simulink model "inverted_pendulum"  (R2021a)
settings: Solver=VariableStepAuto  StartTime=0.0  StopTime=20  MaxStep=0.01  RelTol=1e-3
undefined symbols (not defined in the file): A, alpha, B, beta, bm, bp, C_acc, C_acc_double_enc, C_acc_enc, dt, g, ideal_acc_height, J1, Jw, K, Ke, Kt, L1, L_acc, L_acc_double_enc, L_acc_enc, La, Ra, real_acc_height, V_nom, wn, x0
(part 1 of 2)
settings Model: Creator=jpss8  LastModifiedBy=jpss8

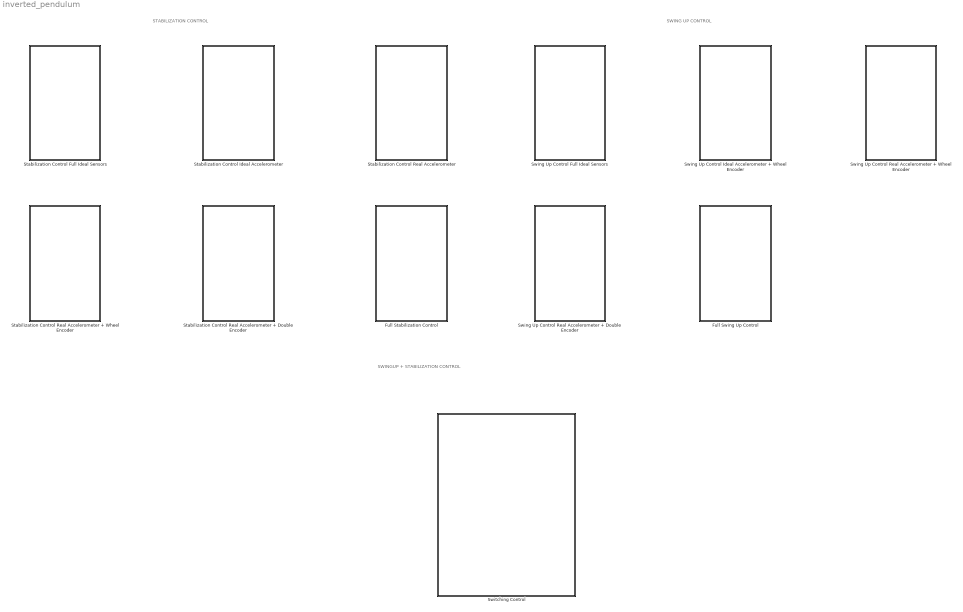
== system inverted_pendulum ==
  note: STABILIZATION CONTROL
  note: SWING UP CONTROL
  note: SWINGUP + STABILIZATION CONTROL
  Full Stabilization Control : Subsystem
  Full Swing Up Control : Subsystem
  Stabilization Control Full Ideal Sensors : Subsystem
  "Stabilization Control Ideal Accelerometer " : Subsystem
  Stabilization Control Real Accelerometer : Subsystem
  Stabilization Control Real Accelerometer + Double Encoder : Subsystem
  Stabilization Control Real Accelerometer + Wheel Encoder : Subsystem
  Swing Up Control Full Ideal Sensors : Subsystem
  Swing Up Control Ideal Accelerometer + Wheel Encoder : Subsystem
  Swing Up Control Real Accelerometer + Double Encoder : Subsystem
  Swing Up Control Real Accelerometer + Wheel Encoder : Subsystem
  Switching Control : Subsystem

== system inverted_pendulum/Full Stabilization Control ==
  note: DC Motor Saturation
  LQR Controller : Subsystem
  Nonlinear Inverted Pendulum : Subsystem
  Real Sensors : Subsystem
  Signal Processing : Subsystem
  State Estimation : Subsystem
  Vmax = 24V : Saturate  UpperLimit=V_nom  LowerLimit=-V_nom
  wires:
  Vmax = 24V/1 -> Nonlinear Inverted Pendulum/1(V), State Estimation/1(V)
  LQR Controller/1(V) -> Vmax = 24V/1
  Real Sensors/1(Acc) -> Signal Processing/4(Acc)
  Real Sensors/2(Gyro) -> Signal Processing/3(Gyro)
  Signal Processing/1(Measured States) -> State Estimation/2(Measured States)
  Nonlinear Inverted Pendulum/1(NL Full State + d2theta) -> Real Sensors/1(NL Full State + d2theta)
  Real Sensors/3(wm) -> Signal Processing/2(wm)
  Real Sensors/4(wp) -> Signal Processing/1(wp)

== system inverted_pendulum/Full Swing Up Control ==
  note: DC Motor Saturation
  Bang Bang Energy Controller : Subsystem
  Ideal Sensors : Subsystem
  Nonlinear Inverted Pendulum : Subsystem
  Vmax = 24V : Saturate  UpperLimit=V_nom  LowerLimit=-V_nom
  wires:
  Vmax = 24V/1 -> Nonlinear Inverted Pendulum/1(V)
  Bang Bang Energy Controller/1(V) -> Vmax = 24V/1
  Nonlinear Inverted Pendulum/1(NL Full State) -> Ideal Sensors/1(Full State)

== system inverted_pendulum/Stabilization Control Full Ideal Sensors ==
  note: DC Motor Saturation
  Ideal Sensors : Subsystem
  LQR Controller : Subsystem
  Nonlinear Inverted Pendulum : Subsystem
  Scope : Scope
  Vmax = 24V : Saturate  UpperLimit=V_nom  LowerLimit=-V_nom
  wires:
  Vmax = 24V/1 -> Nonlinear Inverted Pendulum/1(V)
  LQR Controller/1(V) -> Vmax = 24V/1
  Nonlinear Inverted Pendulum/1(NL Full State) -> Scope/1, Ideal Sensors/1(Full State)
  Ideal Sensors/1(Measured States) -> LQR Controller/1(Measured Full State)

== system inverted_pendulum/Stabilization Control Ideal Accelerometer  ==
  note: DC Motor Saturation
  LQR Controller : Subsystem
  Nonlinear Inverted Pendulum : Subsystem
  Sensors : Subsystem
  Signal Processing : Subsystem
  State Estimation : Subsystem
  Vmax = 24V : Saturate  UpperLimit=V_nom  LowerLimit=-V_nom
  wires:
  Vmax = 24V/1 -> Nonlinear Inverted Pendulum/1(V), State Estimation/1(V)
  LQR Controller/1(V) -> Vmax = 24V/1
  Sensors/1(Acc) -> Signal Processing/1(Acc)
  Signal Processing/1(Measured States) -> State Estimation/2(Measured States)
  Nonlinear Inverted Pendulum/1(NL Full State + d2theta) -> Sensors/1(NL Full State)

== system inverted_pendulum/Stabilization Control Real Accelerometer ==
  note: DC Motor Saturation
  LQR Controller : Subsystem
  Nonlinear Inverted Pendulum : Subsystem
  Sensors : Subsystem
  Signal Processing1 : Subsystem
  State Estimation : Subsystem
  Vmax = 24V : Saturate  UpperLimit=V_nom  LowerLimit=-V_nom
  wires:
  Vmax = 24V/1 -> Nonlinear Inverted Pendulum/1(V), State Estimation/1(V)
  LQR Controller/1(V) -> Vmax = 24V/1
  Sensors/1(Acc) -> Signal Processing1/2(Acc)
  Signal Processing1/1(Measured States) -> State Estimation/2(Measured States)
  Nonlinear Inverted Pendulum/1(NL Full State + d2theta) -> Sensors/1(NL Full State)
  Sensors/2(Gyro) -> Signal Processing1/1(Gyro)

== system inverted_pendulum/Stabilization Control Real Accelerometer + Double Encoder ==
  note: DC Motor Saturation
  LQR Controller : Subsystem
  Nonlinear Inverted Pendulum : Subsystem
  Real Sensors : Subsystem
  Signal Processing : Subsystem
  State Estimation : Subsystem
  Vmax = 24V : Saturate  UpperLimit=V_nom  LowerLimit=-V_nom
  wires:
  Vmax = 24V/1 -> Nonlinear Inverted Pendulum/1(V), State Estimation/1(V)
  LQR Controller/1(V) -> Vmax = 24V/1
  Real Sensors/1(Acc) -> Signal Processing/4(Acc)
  Real Sensors/2(Gyro) -> Signal Processing/3(Gyro)
  Signal Processing/1(Measured States) -> State Estimation/2(Measured States)
  Nonlinear Inverted Pendulum/1(NL Full State + d2theta) -> Real Sensors/1(NL Full State + d2theta)
  Real Sensors/3(wm) -> Signal Processing/2(wm)
  Real Sensors/4(wp) -> Signal Processing/1(wp)

== system inverted_pendulum/Stabilization Control Real Accelerometer + Wheel Encoder ==
  note: DC Motor Saturation
  LQR Controller : Subsystem
  Nonlinear Inverted Pendulum : Subsystem
  Real Sensors : Subsystem
  Signal Processing : Subsystem
  State Estimation : Subsystem
  Vmax = 24V : Saturate  UpperLimit=V_nom  LowerLimit=-V_nom
  wires:
  Vmax = 24V/1 -> Nonlinear Inverted Pendulum/1(V), State Estimation/1(V)
  LQR Controller/1(V) -> Vmax = 24V/1
  Real Sensors/1(Acc) -> Signal Processing/3(Acc)
  Real Sensors/2(Gyro) -> Signal Processing/2(Gyro)
  Signal Processing/1(Measured States) -> State Estimation/2(Measured States)
  Nonlinear Inverted Pendulum/1(NL Full State + d2theta) -> Real Sensors/1(NL Full State)
  Real Sensors/3(wm) -> Signal Processing/1(wm)

== system inverted_pendulum/Swing Up Control Full Ideal Sensors ==
  note: DC Motor Saturation
  Bang Bang Energy Controller : Subsystem
  Demux : Demux
  Ideal Sensors : Subsystem
  Nonlinear Inverted Pendulum : Subsystem
  Scope : Scope
  Scope1 : Scope
  Scope2 : Scope
  Vmax = 24V : Saturate  UpperLimit=V_nom  LowerLimit=-V_nom
  wires:
  Vmax = 24V/1 -> Scope2/1, Nonlinear Inverted Pendulum/1(V)
  Bang Bang Energy Controller/1(V) -> Vmax = 24V/1
  Nonlinear Inverted Pendulum/1(NL Full State) -> Demux/1, Ideal Sensors/1(Full State)
  Demux/1 -> Scope/1
  Demux/3 -> Scope1/1

== system inverted_pendulum/Swing Up Control Ideal Accelerometer + Wheel Encoder ==
  note: DC Motor Saturation
  Bang Bang Energy Controller : Subsystem
  Ideal Sensors : Subsystem
  Nonlinear Inverted Pendulum : Subsystem
  Vmax = 24V : Saturate  UpperLimit=V_nom  LowerLimit=-V_nom
  wires:
  Vmax = 24V/1 -> Nonlinear Inverted Pendulum/1(V)
  Bang Bang Energy Controller/1(V) -> Vmax = 24V/1
  Nonlinear Inverted Pendulum/1(NL Full State) -> Ideal Sensors/1(Full State)

== system inverted_pendulum/Swing Up Control Real Accelerometer + Double Encoder ==
  note: DC Motor Saturation
  Bang Bang Energy Controller : Subsystem
  Ideal Sensors : Subsystem
  Nonlinear Inverted Pendulum : Subsystem
  Vmax = 24V : Saturate  UpperLimit=V_nom  LowerLimit=-V_nom
  wires:
  Vmax = 24V/1 -> Nonlinear Inverted Pendulum/1(V)
  Bang Bang Energy Controller/1(V) -> Vmax = 24V/1
  Nonlinear Inverted Pendulum/1(NL Full State) -> Ideal Sensors/1(Full State)

== system inverted_pendulum/Swing Up Control Real Accelerometer + Wheel Encoder ==
  note: DC Motor Saturation
  Bang Bang Energy Controller : Subsystem
  Ideal Sensors : Subsystem
  Nonlinear Inverted Pendulum : Subsystem
  Vmax = 24V : Saturate  UpperLimit=V_nom  LowerLimit=-V_nom
  wires:
  Vmax = 24V/1 -> Nonlinear Inverted Pendulum/1(V)
  Bang Bang Energy Controller/1(V) -> Vmax = 24V/1
  Nonlinear Inverted Pendulum/1(NL Full State) -> Ideal Sensors/1(Full State)

== system inverted_pendulum/Switching Control ==
  note: DC Motor Saturation
  Constant : Constant  Value=0.25
  Demux : Demux
  Demux1 : Demux
  Ideal Sensors : Subsystem
  Nonlinear Inverted Pendulum : Subsystem
  Scope : Scope  NumInputPorts=2
  Scope1 : Scope
  Switching Controller : Stateflow chart  TreatAsAtomicUnit=on
  Vmax = 24V : Saturate  UpperLimit=V_nom  LowerLimit=-V_nom
  wires:
  Vmax = 24V/1 -> Nonlinear Inverted Pendulum/1(V)
  Nonlinear Inverted Pendulum/1(NL Full State) -> Demux1/1, Ideal Sensors/1(Full State)
  Switching Controller/1(V) -> Vmax = 24V/1
  Demux/1 -> Switching Controller/1(theta)
  Demux/2 -> Switching Controller/2(wp)
  Demux/3 -> Switching Controller/3(wm)
  Demux/4 -> Switching Controller/4(ia)
  Demux1/1 -> Scope/1
  Constant/1 -> Scope/2
  Demux1/3 -> Scope1/1
  Ideal Sensors/1(Measured States) -> Demux/1

== system inverted_pendulum/Full Stabilization Control/LQR Controller ==
  Estimated Full State : Inport
  Gain : Gain  Gain=-K  Multiplication=Matrix(K*u)
  V : Outport
  wires:
  Estimated Full State/1 -> Gain/1
  Gain/1 -> V/1

== system inverted_pendulum/Full Stabilization Control/Nonlinear Inverted Pendulum ==
  V : Inport
  DC Motor + Wheel : Subsystem
  Inverted Pendulum : Subsystem
  Mux : Mux  Inputs=5
  NL Full State + d2theta : Outport
  wires:
  Mux/1 -> NL Full State + d2theta/1
  Inverted Pendulum/3(d2theta) -> Mux/5  "d2theta"
  Inverted Pendulum/2(wp) -> Mux/2  "wp"
  Inverted Pendulum/1(theta) -> Mux/1  "theta"
  DC Motor + Wheel/1(wm) -> Mux/3, Inverted Pendulum/1(wm)  "wm"
  DC Motor + Wheel/2(ia) -> Inverted Pendulum/2(ia), Mux/4  "ia"
  V/1 -> DC Motor + Wheel/1(V)

== system inverted_pendulum/Full Stabilization Control/Real Sensors ==
  NL Full State + d2theta : Inport
  Demux : Demux  Outputs=5
  IMU : Subsystem
  Pendulum Encoder : Subsystem
  Terminator : Terminator
  Wheel Encoder : Subsystem
  Acc : Outport
  Gyro : Outport  Port=2
  wm : Outport  Port=3
  wp : Outport  Port=4
  wires:
  NL Full State + d2theta/1 -> Demux/1
  Demux/1 -> IMU/1(theta)
  Demux/3 -> Wheel Encoder/1(In1)
  Demux/4 -> Terminator/1
  IMU/2(G) -> Gyro/1
  IMU/1(A) -> Acc/1
  Demux/5 -> IMU/3(d2theta)
  Wheel Encoder/1(wm) -> wm/1
  Pendulum Encoder/1(wp) -> wp/1
  Demux/2 -> IMU/2(wp), Pendulum Encoder/1(In1)

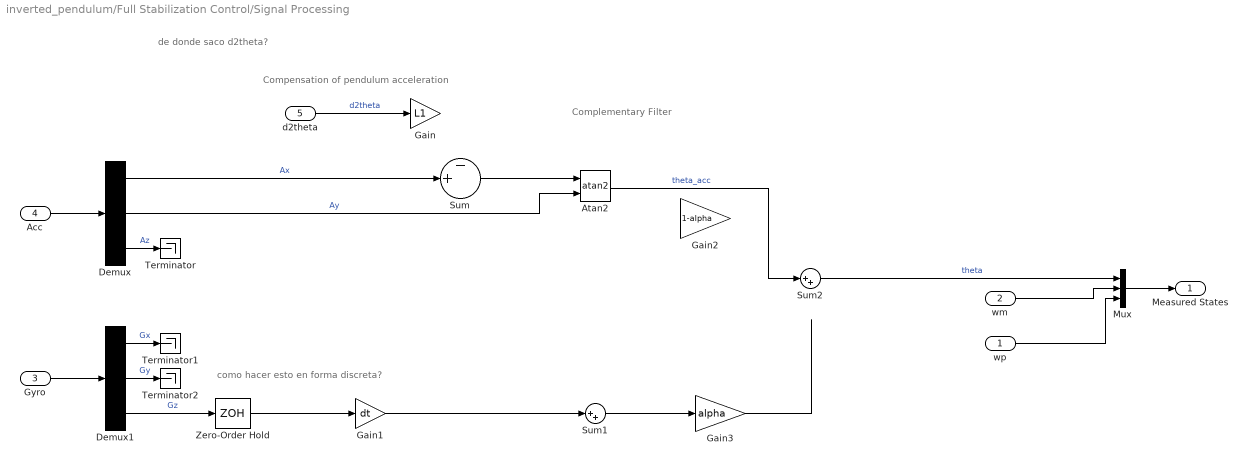
== system inverted_pendulum/Full Stabilization Control/Signal Processing ==
  note: como hacer esto en forma discreta?
  note: Complementary Filter
  note: de donde saco d2theta?
  note: Compensation of pendulum acceleration
  wp : Inport
  wm : Inport  Port=2
  Gyro : Inport  Port=3
  Acc : Inport  Port=4
  d2theta : Inport  Port=5
  Atan2 : Trigonometry  Operator=atan2
  Demux : Demux  Outputs=3
  Demux1 : Demux  Outputs=3
  Gain : Gain  Gain=L1
  Gain1 : Gain  Gain=dt
  Gain2 : Gain  Gain=1-alpha
  Gain3 : Gain  Gain=alpha
  Mux : Mux  Inputs=3
  Sum : Sum  Inputs=-+|
  Sum1 : Sum  Inputs=|++
  Sum2 : Sum  Inputs=|++
  Terminator : Terminator
  Terminator1 : Terminator
  Terminator2 : Terminator
  Zero-Order Hold : ZeroOrderHold  SampleTime=-1
  Measured States : Outport
  wires:
  Gyro/1 -> Demux1/1
  Acc/1 -> Demux/1
  Demux/1 -> Sum/2  "Ax"
  Demux/2 -> Atan2/2  "Ay"
  Demux/3 -> Terminator/1  "Az"
  Sum/1 -> Atan2/1
  d2theta/1 -> Gain/1  "d2theta"
  Atan2/1 -> Sum2/1  "theta_acc"
  Demux1/1 -> Terminator1/1  "Gx"
  Demux1/2 -> Terminator2/1  "Gy"
  Demux1/3 -> Zero-Order Hold/1  "Gz"
  Sum2/1 -> Mux/1  "theta"
  Sum1/1 -> Gain3/1
  Gain1/1 -> Sum1/1
  Zero-Order Hold/1 -> Gain1/1
  Gain3/1 -> ?
  ? -> Sum1/2
  wm/1 -> Mux/2
  Mux/1 -> Measured States/1
  wp/1 -> Mux/3

== system inverted_pendulum/Full Stabilization Control/State Estimation ==
  V : Inport
  Measured States : Inport  Port=2
  Gain : Gain  Gain=L_acc_double_enc  Multiplication=Matrix(K*u)
  Gain1 : Gain  Gain=C_acc_double_enc  Multiplication=Matrix(K*u)
  Gain2 : Gain  Gain=A  Multiplication=Matrix(K*u)
  Gain3 : Gain  Gain=B  Multiplication=Matrix(K*u)
  Integrator : Integrator
  Sum : Sum  Inputs=|+-
  Sum1 : Sum  Inputs=+++
  Estimated Full State : Outport
  wires:
  Measured States/1 -> Sum/1
  V/1 -> Gain3/1
  Integrator/1 -> Gain1/1, Gain2/1, Estimated Full State/1
  Gain3/1 -> Sum1/2
  Sum1/1 -> Integrator/1
  Gain2/1 -> Sum1/3
  Sum/1 -> Gain/1
  Gain1/1 -> Sum/2
  Gain/1 -> Sum1/1

== system inverted_pendulum/Full Swing Up Control/Bang Bang Energy Controller ==
  Measured Full State : Inport
  Demux : Demux
  Energy Calculation : Subsystem
  Gain : Gain  Gain=3.5
  Gain1 : Gain  Gain=0.5
  Gain2 : Gain  Gain=-V_nom
  Product : Product
  Scope : Scope
  Scope1 : Scope
  Sum : Sum  Inputs=|+-
  V : Outport
  wires:
  Energy Calculation/1(Eref-E) -> Scope/1, Product/1
  Measured Full State/1 -> Demux/1
  Demux/2 -> Energy Calculation/2(wp), Product/2  "wp"
  Product/1 -> Gain/1
  Gain/1 -> Sum/1
  Demux/3 -> Gain1/1  "wm"
  Gain1/1 -> Sum/2
  Sum/1 -> Gain2/1
  Demux/1 -> Energy Calculation/1(theta)
  Gain2/1 -> Scope1/1, V/1

== system inverted_pendulum/Full Swing Up Control/Ideal Sensors ==
  note: Ideal Sensors
  Full State : Inport
  Gain : Gain
  Measured States : Outport
  wires:
  Full State/1 -> Gain/1
  Gain/1 -> Measured States/1

== system inverted_pendulum/Full Swing Up Control/Nonlinear Inverted Pendulum ==
  V : Inport
  DC Motor + Wheel : Subsystem
  Inverted Pendulum : Subsystem
  Mux : Mux
  NL Full State : Outport
  wires:
  Mux/1 -> NL Full State/1
  Inverted Pendulum/2(wp) -> Mux/2  "wp"
  Inverted Pendulum/1(theta) -> Mux/1  "theta"
  DC Motor + Wheel/1(wm) -> Mux/3, Inverted Pendulum/1(wm)  "wm"
  DC Motor + Wheel/2(ia) -> Inverted Pendulum/2(ia), Mux/4  "ia"
  V/1 -> DC Motor + Wheel/1(V)

== system inverted_pendulum/Stabilization Control Full Ideal Sensors/Ideal Sensors ==
  note: Ideal Sensors
  Full State : Inport
  Gain : Gain
  Measured States : Outport
  wires:
  Full State/1 -> Gain/1
  Gain/1 -> Measured States/1

== system inverted_pendulum/Stabilization Control Full Ideal Sensors/LQR Controller ==
  Measured Full State : Inport
  Gain : Gain  Gain=-K  Multiplication=Matrix(K*u)
  V : Outport
  wires:
  Measured Full State/1 -> Gain/1
  Gain/1 -> V/1

== system inverted_pendulum/Stabilization Control Full Ideal Sensors/Nonlinear Inverted Pendulum ==
  V : Inport
  DC Motor + Wheel : Subsystem
  Inverted Pendulum : Subsystem
  Mux : Mux
  NL Full State : Outport
  wires:
  Mux/1 -> NL Full State/1
  Inverted Pendulum/2(wp) -> Mux/2  "wp"
  Inverted Pendulum/1(theta) -> Mux/1  "theta"
  DC Motor + Wheel/1(wm) -> Mux/3, Inverted Pendulum/1(wm)  "wm"
  DC Motor + Wheel/2(ia) -> Inverted Pendulum/2(ia), Mux/4  "ia"
  V/1 -> DC Motor + Wheel/1(V)

== system inverted_pendulum/Stabilization Control Ideal Accelerometer /LQR Controller ==
  Estimated Full State : Inport
  Gain : Gain  Gain=-K  Multiplication=Matrix(K*u)
  V : Outport
  wires:
  Estimated Full State/1 -> Gain/1
  Gain/1 -> V/1

== system inverted_pendulum/Stabilization Control Ideal Accelerometer /Nonlinear Inverted Pendulum ==
  V : Inport
  DC Motor + Wheel : Subsystem
  Inverted Pendulum : Subsystem
  Mux : Mux  Inputs=5
  NL Full State + d2theta : Outport
  wires:
  Mux/1 -> NL Full State + d2theta/1
  Inverted Pendulum/3(d2theta) -> Mux/5  "d2theta"
  Inverted Pendulum/2(wp) -> Mux/2  "wp"
  Inverted Pendulum/1(theta) -> Mux/1  "theta"
  DC Motor + Wheel/1(wm) -> Mux/3, Inverted Pendulum/1(wm)  "wm"
  DC Motor + Wheel/2(ia) -> Inverted Pendulum/2(ia), Mux/4  "ia"
  V/1 -> DC Motor + Wheel/1(V)

== system inverted_pendulum/Stabilization Control Ideal Accelerometer /Sensors ==
  NL Full State : Inport
  Demux : Demux  Outputs=5
  IMU : Subsystem
  Terminator : Terminator
  Terminator1 : Terminator
  Acc : Outport
  Gyro : Outport  Port=2
  wires:
  NL Full State/1 -> Demux/1
  Demux/2 -> IMU/2(wp)
  Demux/1 -> IMU/1(theta)
  Demux/4 -> Terminator/1
  IMU/2(G) -> Gyro/1
  IMU/1(A) -> Acc/1
  Demux/5 -> IMU/3(d2theta)
  Demux/3 -> Terminator1/1

== system inverted_pendulum/Stabilization Control Ideal Accelerometer /Signal Processing ==
  Acc : Inport
  Atan2 : Trigonometry  Operator=atan2
  Demux : Demux  Outputs=3
  Terminator : Terminator
  Measured States : Outport
  wires:
  Acc/1 -> Demux/1
  Demux/1 -> Atan2/1  "Ax"
  Demux/2 -> Atan2/2  "Ay"
  Demux/3 -> Terminator/1  "Az"
  Atan2/1 -> Measured States/1  "theta_acc"

== system inverted_pendulum/Stabilization Control Ideal Accelerometer /State Estimation ==
  V : Inport
  Measured States : Inport  Port=2
  Gain : Gain  Gain=L_acc  Multiplication=Matrix(K*u)
  Gain1 : Gain  Gain=C_acc  Multiplication=Matrix(K*u)
  Gain2 : Gain  Gain=A  Multiplication=Matrix(K*u)
  Gain3 : Gain  Gain=B  Multiplication=Matrix(K*u)
  Integrator : Integrator
  Sum : Sum  Inputs=|+-
  Sum1 : Sum  Inputs=+++
  Estimated Full State : Outport
  wires:
  Measured States/1 -> Sum/1
  V/1 -> Gain3/1
  Integrator/1 -> Gain1/1, Gain2/1, Estimated Full State/1
  Gain3/1 -> Sum1/2
  Sum1/1 -> Integrator/1
  Gain2/1 -> Sum1/3
  Sum/1 -> Gain/1
  Gain1/1 -> Sum/2
  Gain/1 -> Sum1/1

== system inverted_pendulum/Stabilization Control Real Accelerometer/LQR Controller ==
  Estimated Full State : Inport
  Gain : Gain  Gain=-K  Multiplication=Matrix(K*u)
  V : Outport
  wires:
  Estimated Full State/1 -> Gain/1
  Gain/1 -> V/1

== system inverted_pendulum/Stabilization Control Real Accelerometer/Nonlinear Inverted Pendulum ==
  V : Inport
  DC Motor + Wheel : Subsystem
  Inverted Pendulum : Subsystem
  Mux : Mux  Inputs=5
  NL Full State + d2theta : Outport
  wires:
  Mux/1 -> NL Full State + d2theta/1
  Inverted Pendulum/3(d2theta) -> Mux/5  "d2theta"
  Inverted Pendulum/2(wp) -> Mux/2  "wp"
  Inverted Pendulum/1(theta) -> Mux/1  "theta"
  DC Motor + Wheel/1(wm) -> Mux/3, Inverted Pendulum/1(wm)  "wm"
  DC Motor + Wheel/2(ia) -> Inverted Pendulum/2(ia), Mux/4  "ia"
  V/1 -> DC Motor + Wheel/1(V)

== system inverted_pendulum/Stabilization Control Real Accelerometer/Sensors ==
  NL Full State : Inport
  Demux : Demux  Outputs=5
  IMU : Subsystem
  Terminator : Terminator
  Terminator1 : Terminator
  Acc : Outport
  Gyro : Outport  Port=2
  wires:
  NL Full State/1 -> Demux/1
  Demux/2 -> IMU/2(wp)
  Demux/1 -> IMU/1(theta)
  Demux/4 -> Terminator/1
  IMU/2(G) -> Gyro/1
  IMU/1(A) -> Acc/1
  Demux/5 -> IMU/3(d2theta)
  Demux/3 -> Terminator1/1

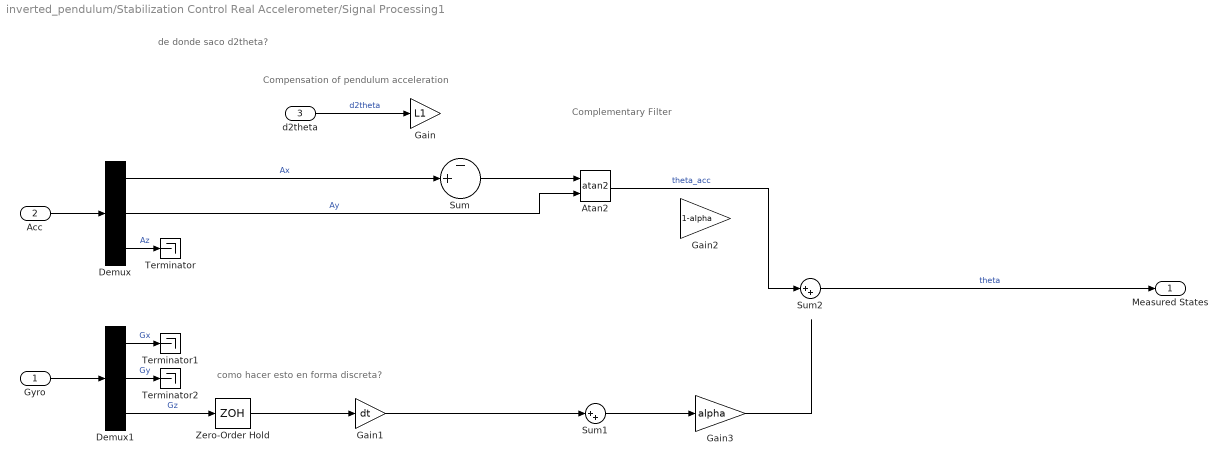
== system inverted_pendulum/Stabilization Control Real Accelerometer/Signal Processing1 ==
  note: como hacer esto en forma discreta?
  note: Complementary Filter
  note: de donde saco d2theta?
  note: Compensation of pendulum acceleration
  Gyro : Inport
  Acc : Inport  Port=2
  d2theta : Inport  Port=3
  Atan2 : Trigonometry  Operator=atan2
  Demux : Demux  Outputs=3
  Demux1 : Demux  Outputs=3
  Gain : Gain  Gain=L1
  Gain1 : Gain  Gain=dt
  Gain2 : Gain  Gain=1-alpha
  Gain3 : Gain  Gain=alpha
  Sum : Sum  Inputs=-+|
  Sum1 : Sum  Inputs=|++
  Sum2 : Sum  Inputs=|++
  Terminator : Terminator
  Terminator1 : Terminator
  Terminator2 : Terminator
  Zero-Order Hold : ZeroOrderHold  SampleTime=-1
  Measured States : Outport
  wires:
  Gyro/1 -> Demux1/1
  Acc/1 -> Demux/1
  Demux/1 -> Sum/2  "Ax"
  Demux/2 -> Atan2/2  "Ay"
  Demux/3 -> Terminator/1  "Az"
  Sum/1 -> Atan2/1
  d2theta/1 -> Gain/1  "d2theta"
  Atan2/1 -> Sum2/1  "theta_acc"
  Demux1/1 -> Terminator1/1  "Gx"
  Demux1/2 -> Terminator2/1  "Gy"
  Demux1/3 -> Zero-Order Hold/1  "Gz"
  Sum2/1 -> Measured States/1  "theta"
  Sum1/1 -> Gain3/1
  Gain1/1 -> Sum1/1
  Zero-Order Hold/1 -> Gain1/1
  Gain3/1 -> ?
  ? -> Sum1/2

== system inverted_pendulum/Stabilization Control Real Accelerometer/State Estimation ==
  V : Inport
  Measured States : Inport  Port=2
  Gain : Gain  Gain=L_acc  Multiplication=Matrix(K*u)
  Gain1 : Gain  Gain=C_acc  Multiplication=Matrix(K*u)
  Gain2 : Gain  Gain=A  Multiplication=Matrix(K*u)
  Gain3 : Gain  Gain=B  Multiplication=Matrix(K*u)
  Integrator : Integrator
  Sum : Sum  Inputs=|+-
  Sum1 : Sum  Inputs=+++
  Estimated Full State : Outport
  wires:
  Measured States/1 -> Sum/1
  V/1 -> Gain3/1
  Integrator/1 -> Gain1/1, Gain2/1, Estimated Full State/1
  Gain3/1 -> Sum1/2
  Sum1/1 -> Integrator/1
  Gain2/1 -> Sum1/3
  Sum/1 -> Gain/1
  Gain1/1 -> Sum/2
  Gain/1 -> Sum1/1

== system inverted_pendulum/Stabilization Control Real Accelerometer + Double Encoder/LQR Controller ==
  Estimated Full State : Inport
  Gain : Gain  Gain=-K  Multiplication=Matrix(K*u)
  V : Outport
  wires:
  Estimated Full State/1 -> Gain/1
  Gain/1 -> V/1

== system inverted_pendulum/Stabilization Control Real Accelerometer + Double Encoder/Nonlinear Inverted Pendulum ==
  V : Inport
  DC Motor + Wheel : Subsystem
  Inverted Pendulum : Subsystem
  Mux : Mux  Inputs=5
  NL Full State + d2theta : Outport
  wires:
  Mux/1 -> NL Full State + d2theta/1
  Inverted Pendulum/3(d2theta) -> Mux/5  "d2theta"
  Inverted Pendulum/2(wp) -> Mux/2  "wp"
  Inverted Pendulum/1(theta) -> Mux/1  "theta"
  DC Motor + Wheel/1(wm) -> Mux/3, Inverted Pendulum/1(wm)  "wm"
  DC Motor + Wheel/2(ia) -> Inverted Pendulum/2(ia), Mux/4  "ia"
  V/1 -> DC Motor + Wheel/1(V)

== system inverted_pendulum/Stabilization Control Real Accelerometer + Double Encoder/Real Sensors ==
  NL Full State + d2theta : Inport
  Demux : Demux  Outputs=5
  IMU : Subsystem
  Pendulum Encoder : Subsystem
  Terminator : Terminator
  Wheel Encoder : Subsystem
  Acc : Outport
  Gyro : Outport  Port=2
  wm : Outport  Port=3
  wp : Outport  Port=4
  wires:
  NL Full State + d2theta/1 -> Demux/1
  Demux/1 -> IMU/1(theta)
  Demux/3 -> Wheel Encoder/1(In1)
  Demux/4 -> Terminator/1
  IMU/2(G) -> Gyro/1
  IMU/1(A) -> Acc/1
  Demux/5 -> IMU/3(d2theta)
  Wheel Encoder/1(wm) -> wm/1
  Pendulum Encoder/1(wp) -> wp/1
  Demux/2 -> IMU/2(wp), Pendulum Encoder/1(In1)

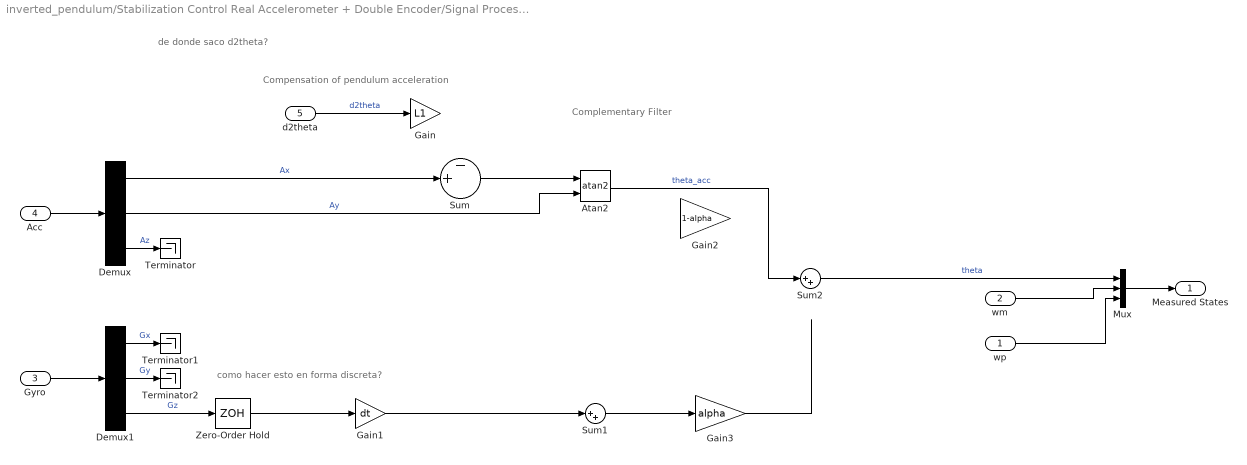
== system inverted_pendulum/Stabilization Control Real Accelerometer + Double Encoder/Signal Processing ==
  note: como hacer esto en forma discreta?
  note: Complementary Filter
  note: de donde saco d2theta?
  note: Compensation of pendulum acceleration
  wp : Inport
  wm : Inport  Port=2
  Gyro : Inport  Port=3
  Acc : Inport  Port=4
  d2theta : Inport  Port=5
  Atan2 : Trigonometry  Operator=atan2
  Demux : Demux  Outputs=3
  Demux1 : Demux  Outputs=3
  Gain : Gain  Gain=L1
  Gain1 : Gain  Gain=dt
  Gain2 : Gain  Gain=1-alpha
  Gain3 : Gain  Gain=alpha
  Mux : Mux  Inputs=3
  Sum : Sum  Inputs=-+|
  Sum1 : Sum  Inputs=|++
  Sum2 : Sum  Inputs=|++
  Terminator : Terminator
  Terminator1 : Terminator
  Terminator2 : Terminator
  Zero-Order Hold : ZeroOrderHold  SampleTime=-1
  Measured States : Outport
  wires:
  Gyro/1 -> Demux1/1
  Acc/1 -> Demux/1
  Demux/1 -> Sum/2  "Ax"
  Demux/2 -> Atan2/2  "Ay"
  Demux/3 -> Terminator/1  "Az"
  Sum/1 -> Atan2/1
  d2theta/1 -> Gain/1  "d2theta"
  Atan2/1 -> Sum2/1  "theta_acc"
  Demux1/1 -> Terminator1/1  "Gx"
  Demux1/2 -> Terminator2/1  "Gy"
  Demux1/3 -> Zero-Order Hold/1  "Gz"
  Sum2/1 -> Mux/1  "theta"
  Sum1/1 -> Gain3/1
  Gain1/1 -> Sum1/1
  Zero-Order Hold/1 -> Gain1/1
  Gain3/1 -> ?
  ? -> Sum1/2
  wm/1 -> Mux/2
  Mux/1 -> Measured States/1
  wp/1 -> Mux/3

== system inverted_pendulum/Stabilization Control Real Accelerometer + Double Encoder/State Estimation ==
  V : Inport
  Measured States : Inport  Port=2
  Gain : Gain  Gain=L_acc_double_enc  Multiplication=Matrix(K*u)
  Gain1 : Gain  Gain=C_acc_double_enc  Multiplication=Matrix(K*u)
  Gain2 : Gain  Gain=A  Multiplication=Matrix(K*u)
  Gain3 : Gain  Gain=B  Multiplication=Matrix(K*u)
  Integrator : Integrator
  Sum : Sum  Inputs=|+-
  Sum1 : Sum  Inputs=+++
  Estimated Full State : Outport
  wires:
  Measured States/1 -> Sum/1
  V/1 -> Gain3/1
  Integrator/1 -> Gain1/1, Gain2/1, Estimated Full State/1
  Gain3/1 -> Sum1/2
  Sum1/1 -> Integrator/1
  Gain2/1 -> Sum1/3
  Sum/1 -> Gain/1
  Gain1/1 -> Sum/2
  Gain/1 -> Sum1/1

== system inverted_pendulum/Stabilization Control Real Accelerometer + Wheel Encoder/LQR Controller ==
  Estimated Full State : Inport
  Gain : Gain  Gain=-K  Multiplication=Matrix(K*u)
  V : Outport
  wires:
  Estimated Full State/1 -> Gain/1
  Gain/1 -> V/1

== system inverted_pendulum/Stabilization Control Real Accelerometer + Wheel Encoder/Nonlinear Inverted Pendulum ==
  V : Inport
  DC Motor + Wheel : Subsystem
  Inverted Pendulum : Subsystem
  Mux : Mux  Inputs=5
  NL Full State + d2theta : Outport
  wires:
  Mux/1 -> NL Full State + d2theta/1
  Inverted Pendulum/3(d2theta) -> Mux/5  "d2theta"
  Inverted Pendulum/2(wp) -> Mux/2  "wp"
  Inverted Pendulum/1(theta) -> Mux/1  "theta"
  DC Motor + Wheel/1(wm) -> Mux/3, Inverted Pendulum/1(wm)  "wm"
  DC Motor + Wheel/2(ia) -> Inverted Pendulum/2(ia), Mux/4  "ia"
  V/1 -> DC Motor + Wheel/1(V)

== system inverted_pendulum/Stabilization Control Real Accelerometer + Wheel Encoder/Real Sensors ==
  NL Full State : Inport
  Demux : Demux  Outputs=5
  IMU : Subsystem
  Terminator : Terminator
  Wheel Encoder : Subsystem
  Acc : Outport
  Gyro : Outport  Port=2
  wm : Outport  Port=3
  wires:
  NL Full State/1 -> Demux/1
  Demux/2 -> IMU/2(wp)
  Demux/1 -> IMU/1(theta)
  Demux/3 -> Wheel Encoder/1(In1)
  Demux/4 -> Terminator/1
  IMU/2(G) -> Gyro/1
  IMU/1(A) -> Acc/1
  Demux/5 -> IMU/3(d2theta)
  Wheel Encoder/1(wm) -> wm/1

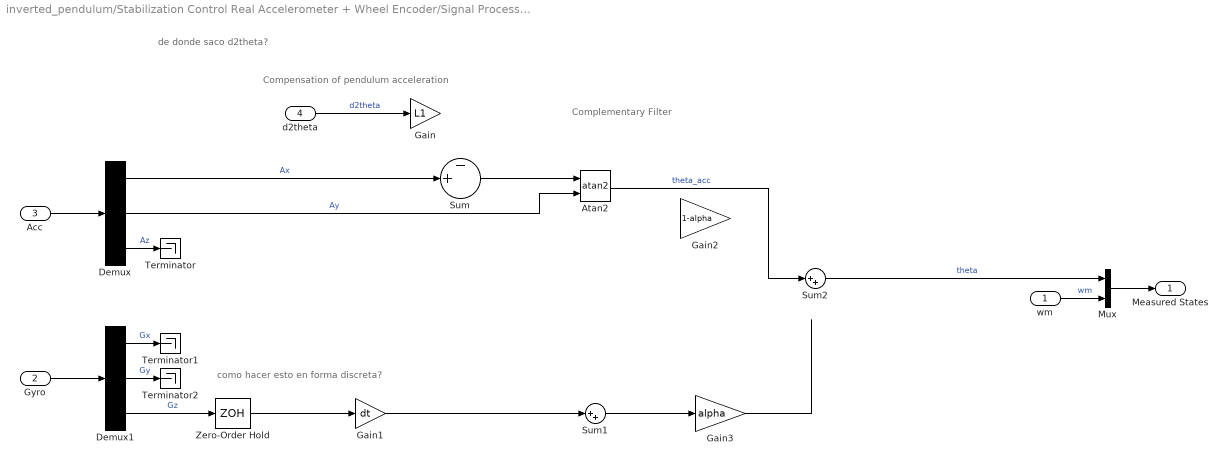
== system inverted_pendulum/Stabilization Control Real Accelerometer + Wheel Encoder/Signal Processing ==
  note: como hacer esto en forma discreta?
  note: Complementary Filter
  note: de donde saco d2theta?
  note: Compensation of pendulum acceleration
  wm : Inport
  Gyro : Inport  Port=2
  Acc : Inport  Port=3
  d2theta : Inport  Port=4
  Atan2 : Trigonometry  Operator=atan2
  Demux : Demux  Outputs=3
  Demux1 : Demux  Outputs=3
  Gain : Gain  Gain=L1
  Gain1 : Gain  Gain=dt
  Gain2 : Gain  Gain=1-alpha
  Gain3 : Gain  Gain=alpha
  Mux : Mux  Inputs=2
  Sum : Sum  Inputs=-+|
  Sum1 : Sum  Inputs=|++
  Sum2 : Sum  Inputs=|++
  Terminator : Terminator
  Terminator1 : Terminator
  Terminator2 : Terminator
  Zero-Order Hold : ZeroOrderHold  SampleTime=-1
  Measured States : Outport
  wires:
  Gyro/1 -> Demux1/1
  Acc/1 -> Demux/1
  Demux/1 -> Sum/2  "Ax"
  Demux/2 -> Atan2/2  "Ay"
  Demux/3 -> Terminator/1  "Az"
  Sum/1 -> Atan2/1
  d2theta/1 -> Gain/1  "d2theta"
  Atan2/1 -> Sum2/1  "theta_acc"
  Demux1/1 -> Terminator1/1  "Gx"
  Demux1/2 -> Terminator2/1  "Gy"
  Demux1/3 -> Zero-Order Hold/1  "Gz"
  Sum2/1 -> Mux/1  "theta"
  Sum1/1 -> Gain3/1
  Gain1/1 -> Sum1/1
  Zero-Order Hold/1 -> Gain1/1
  Gain3/1 -> ?
  ? -> Sum1/2
  Mux/1 -> Measured States/1
  wm/1 -> Mux/2  "wm"

== system inverted_pendulum/Stabilization Control Real Accelerometer + Wheel Encoder/State Estimation ==
  V : Inport
  Measured States : Inport  Port=2
  Gain : Gain  Gain=L_acc_enc  Multiplication=Matrix(K*u)
  Gain1 : Gain  Gain=C_acc_enc  Multiplication=Matrix(K*u)
  Gain2 : Gain  Gain=A  Multiplication=Matrix(K*u)
  Gain3 : Gain  Gain=B  Multiplication=Matrix(K*u)
  Integrator : Integrator
  Sum : Sum  Inputs=|+-
  Sum1 : Sum  Inputs=+++
  Estimated Full State : Outport
  wires:
  Measured States/1 -> Sum/1
  V/1 -> Gain3/1
  Integrator/1 -> Gain1/1, Gain2/1, Estimated Full State/1
  Gain3/1 -> Sum1/2
  Sum1/1 -> Integrator/1
  Gain2/1 -> Sum1/3
  Sum/1 -> Gain/1
  Gain1/1 -> Sum/2
  Gain/1 -> Sum1/1

== system inverted_pendulum/Swing Up Control Full Ideal Sensors/Bang Bang Energy Controller ==
  Measured Full State : Inport
  Demux : Demux
  Energy Calculation : Subsystem
  Gain : Gain
  Gain1 : Gain  Gain=0.17
  Gain2 : Gain  Gain=-V_nom
  Product : Product
  Scope : Scope
  Scope1 : Scope
  Sum : Sum  Inputs=|+-
  V : Outport
  wires:
  Energy Calculation/1(Eref-E) -> Scope/1, Product/1
  Measured Full State/1 -> Demux/1
  Demux/2 -> Energy Calculation/2(wp), Product/2  "wp"
  Product/1 -> Gain/1
  Gain/1 -> Sum/1
  Demux/3 -> Gain1/1  "wm"
  Gain1/1 -> Sum/2
  Sum/1 -> Gain2/1
  Demux/1 -> Energy Calculation/1(theta)
  Gain2/1 -> Scope1/1, V/1

== system inverted_pendulum/Swing Up Control Full Ideal Sensors/Ideal Sensors ==
  note: Ideal Sensors
  Full State : Inport
  Gain : Gain
  Measured States : Outport
  wires:
  Full State/1 -> Gain/1
  Gain/1 -> Measured States/1

== system inverted_pendulum/Swing Up Control Full Ideal Sensors/Nonlinear Inverted Pendulum ==
  V : Inport
  DC Motor + Wheel : Subsystem
  Inverted Pendulum : Subsystem
  Mux : Mux
  NL Full State : Outport
  wires:
  Mux/1 -> NL Full State/1
  Inverted Pendulum/2(wp) -> Mux/2  "wp"
  Inverted Pendulum/1(theta) -> Mux/1  "theta"
  DC Motor + Wheel/1(wm) -> Mux/3, Inverted Pendulum/1(wm)  "wm"
  DC Motor + Wheel/2(ia) -> Inverted Pendulum/2(ia), Mux/4  "ia"
  V/1 -> DC Motor + Wheel/1(V)

== system inverted_pendulum/Swing Up Control Ideal Accelerometer + Wheel Encoder/Bang Bang Energy Controller ==
  Measured Full State : Inport
  Demux : Demux
  Energy Calculation : Subsystem
  Gain : Gain  Gain=3.5
  Gain1 : Gain  Gain=0.5
  Gain2 : Gain  Gain=-V_nom
  Product : Product
  Scope : Scope
  Scope1 : Scope
  Sum : Sum  Inputs=|+-
  V : Outport
  wires:
  Energy Calculation/1(Eref-E) -> Scope/1, Product/1
  Measured Full State/1 -> Demux/1
  Demux/2 -> Energy Calculation/2(wp), Product/2  "wp"
  Product/1 -> Gain/1
  Gain/1 -> Sum/1
  Demux/3 -> Gain1/1  "wm"
  Gain1/1 -> Sum/2
  Sum/1 -> Gain2/1
  Demux/1 -> Energy Calculation/1(theta)
  Gain2/1 -> Scope1/1, V/1

== system inverted_pendulum/Swing Up Control Ideal Accelerometer + Wheel Encoder/Ideal Sensors ==
  note: Ideal Sensors
  Full State : Inport
  Gain : Gain
  Measured States : Outport
  wires:
  Full State/1 -> Gain/1
  Gain/1 -> Measured States/1

== system inverted_pendulum/Swing Up Control Ideal Accelerometer + Wheel Encoder/Nonlinear Inverted Pendulum ==
  V : Inport
  DC Motor + Wheel : Subsystem
  Inverted Pendulum : Subsystem
  Mux : Mux
  NL Full State : Outport
  wires:
  Mux/1 -> NL Full State/1
  Inverted Pendulum/2(wp) -> Mux/2  "wp"
  Inverted Pendulum/1(theta) -> Mux/1  "theta"
  DC Motor + Wheel/1(wm) -> Mux/3, Inverted Pendulum/1(wm)  "wm"
  DC Motor + Wheel/2(ia) -> Inverted Pendulum/2(ia), Mux/4  "ia"
  V/1 -> DC Motor + Wheel/1(V)

== system inverted_pendulum/Swing Up Control Real Accelerometer + Double Encoder/Bang Bang Energy Controller ==
  Measured Full State : Inport
  Demux : Demux
  Energy Calculation : Subsystem
  Gain : Gain  Gain=3.5
  Gain1 : Gain  Gain=0.5
  Gain2 : Gain  Gain=-V_nom
  Product : Product
  Scope : Scope
  Scope1 : Scope
  Sum : Sum  Inputs=|+-
  V : Outport
  wires:
  Energy Calculation/1(Eref-E) -> Scope/1, Product/1
  Measured Full State/1 -> Demux/1
  Demux/2 -> Energy Calculation/2(wp), Product/2  "wp"
  Product/1 -> Gain/1
  Gain/1 -> Sum/1
  Demux/3 -> Gain1/1  "wm"
  Gain1/1 -> Sum/2
  Sum/1 -> Gain2/1
  Demux/1 -> Energy Calculation/1(theta)
  Gain2/1 -> Scope1/1, V/1

== system inverted_pendulum/Swing Up Control Real Accelerometer + Double Encoder/Ideal Sensors ==
  note: Ideal Sensors
  Full State : Inport
  Gain : Gain
  Measured States : Outport
  wires:
  Full State/1 -> Gain/1
  Gain/1 -> Measured States/1

== system inverted_pendulum/Swing Up Control Real Accelerometer + Double Encoder/Nonlinear Inverted Pendulum ==
  V : Inport
  DC Motor + Wheel : Subsystem
  Inverted Pendulum : Subsystem
  Mux : Mux
  NL Full State : Outport
  wires:
  Mux/1 -> NL Full State/1
  Inverted Pendulum/2(wp) -> Mux/2  "wp"
  Inverted Pendulum/1(theta) -> Mux/1  "theta"
  DC Motor + Wheel/1(wm) -> Mux/3, Inverted Pendulum/1(wm)  "wm"
  DC Motor + Wheel/2(ia) -> Inverted Pendulum/2(ia), Mux/4  "ia"
  V/1 -> DC Motor + Wheel/1(V)

== system inverted_pendulum/Swing Up Control Real Accelerometer + Wheel Encoder/Bang Bang Energy Controller ==
  Measured Full State : Inport
  Demux : Demux
  Energy Calculation : Subsystem
  Gain : Gain  Gain=3.5
  Gain1 : Gain  Gain=0.5
  Gain2 : Gain  Gain=-V_nom
  Product : Product
  Scope : Scope
  Scope1 : Scope
  Sum : Sum  Inputs=|+-
  V : Outport
  wires:
  Energy Calculation/1(Eref-E) -> Scope/1, Product/1
  Measured Full State/1 -> Demux/1
  Demux/2 -> Energy Calculation/2(wp), Product/2  "wp"
  Product/1 -> Gain/1
  Gain/1 -> Sum/1
  Demux/3 -> Gain1/1  "wm"
  Gain1/1 -> Sum/2
  Sum/1 -> Gain2/1
  Demux/1 -> Energy Calculation/1(theta)
  Gain2/1 -> Scope1/1, V/1

== system inverted_pendulum/Swing Up Control Real Accelerometer + Wheel Encoder/Ideal Sensors ==
  note: Ideal Sensors
  Full State : Inport
  Gain : Gain
  Measured States : Outport
  wires:
  Full State/1 -> Gain/1
  Gain/1 -> Measured States/1

== system inverted_pendulum/Swing Up Control Real Accelerometer + Wheel Encoder/Nonlinear Inverted Pendulum ==
  V : Inport
  DC Motor + Wheel : Subsystem
  Inverted Pendulum : Subsystem
  Mux : Mux
  NL Full State : Outport
  wires:
  Mux/1 -> NL Full State/1
  Inverted Pendulum/2(wp) -> Mux/2  "wp"
  Inverted Pendulum/1(theta) -> Mux/1  "theta"
  DC Motor + Wheel/1(wm) -> Mux/3, Inverted Pendulum/1(wm)  "wm"
  DC Motor + Wheel/2(ia) -> Inverted Pendulum/2(ia), Mux/4  "ia"
  V/1 -> DC Motor + Wheel/1(V)

== system inverted_pendulum/Switching Control/Ideal Sensors ==
  note: Ideal Sensors
  Full State : Inport
  Gain : Gain
  Measured States : Outport
  wires:
  Full State/1 -> Gain/1
  Gain/1 -> Measured States/1

== system inverted_pendulum/Switching Control/Nonlinear Inverted Pendulum ==
  V : Inport
  DC Motor + Wheel : Subsystem
  Inverted Pendulum : Subsystem
  Mux : Mux
  NL Full State : Outport
  wires:
  Mux/1 -> NL Full State/1
  Inverted Pendulum/2(wp) -> Mux/2  "wp"
  Inverted Pendulum/1(theta) -> Mux/1  "theta"
  DC Motor + Wheel/1(wm) -> Mux/3, Inverted Pendulum/1(wm)  "wm"
  DC Motor + Wheel/2(ia) -> Inverted Pendulum/2(ia), Mux/4  "ia"
  V/1 -> DC Motor + Wheel/1(V)

== system inverted_pendulum/Switching Control/Switching Controller/Stabilization.Stabilization ==
  theta : Inport  OutDataTypeStr=double  PortDimensions=1
  wp : Inport  Port=2  OutDataTypeStr=double  PortDimensions=1
  wm : Inport  Port=3  OutDataTypeStr=double  PortDimensions=1
  ia : Inport  Port=4  OutDataTypeStr=double  PortDimensions=1
  f : TriggerPort  TriggerType=function-call  VariantControl=(inherit)
      settings: CopyFcn=Stateflow.SLINSF.SimulinkMan.removeBlockPreDeleteFcn  PreDeleteFcn=Stateflow.SLINSF.SimulinkMan.unsafePredeleteFcn
  Gain : Gain  Gain=-K  Multiplication=Matrix(K*u)
  Mux : Mux
  V : Outport
  wires:
  Gain/1 -> V/1
  Mux/1 -> Gain/1
  theta/1 -> Mux/1
  wp/1 -> Mux/2
  wm/1 -> Mux/3
  ia/1 -> Mux/4

== system inverted_pendulum/Switching Control/Switching Controller/SwingUp.SwingUp ==
  theta : Inport  OutDataTypeStr=double  PortDimensions=1
  wp : Inport  Port=2  OutDataTypeStr=double  PortDimensions=1
  wm : Inport  Port=3  OutDataTypeStr=double  PortDimensions=1
  ia : Inport  Port=4  OutDataTypeStr=double  PortDimensions=1
  f : TriggerPort  TriggerType=function-call  VariantControl=(inherit)
      settings: CopyFcn=Stateflow.SLINSF.SimulinkMan.removeBlockPreDeleteFcn  PreDeleteFcn=Stateflow.SLINSF.SimulinkMan.unsafePredeleteFcn
  Energy Calculation : Subsystem
  Gain : Gain
  Gain1 : Gain  Gain=0.17
  Gain2 : Gain  Gain=-V_nom
  Product : Product
  Sum : Sum  Inputs=|+-
  Terminator : Terminator
  V : Outport
  wires:
  Gain2/1 -> V/1
  theta/1 -> Energy Calculation/1(theta)
  Sum/1 -> Gain2/1
  wm/1 -> Gain1/1  "wm"
  Gain/1 -> Sum/1
  Gain1/1 -> Sum/2
  Product/1 -> Gain/1
  wp/1 -> Energy Calculation/2(wp), Product/2  "wp"
  Energy Calculation/1(Eref-E) -> Product/1
  ia/1 -> Terminator/1

== system inverted_pendulum/Full Stabilization Control/Nonlinear Inverted Pendulum/DC Motor + Wheel ==
  note: Wheel
  note: DC Motor
  V : Inport
  Gain : Gain  Gain=1/Jw
  Gain1 : Gain  Gain=bm
  Gain2 : Gain  Gain=Kt
  Gain3 : Gain  Gain=1/La
  Gain4 : Gain  Gain=Ra
  Gain5 : Gain  Gain=Ke
  Integrator ia : Integrator  InitialCondition=x0(4)
  Integrator wm : Integrator  InitialCondition=x0(3)
  Sum : Sum  Inputs=|+-
  Sum1 : Sum  Inputs=|+--
  wm : Outport
  ia : Outport  Port=2
  wires:
  Sum/1 -> Gain/1
  Gain/1 -> Integrator wm/1  "d2phi"
  Integrator wm/1 -> wm/1, Gain1/1, Gain5/1  "wm"
  Gain1/1 -> Sum/2
  Gain2/1 -> Sum/1
  Integrator ia/1 -> ia/1, Gain4/1, Gain2/1  "ia"
  Gain3/1 -> Integrator ia/1  "di/dt"
  Sum1/1 -> Gain3/1
  Gain4/1 -> Sum1/3
  V/1 -> Sum1/1  "V"
  Gain5/1 -> Sum1/2

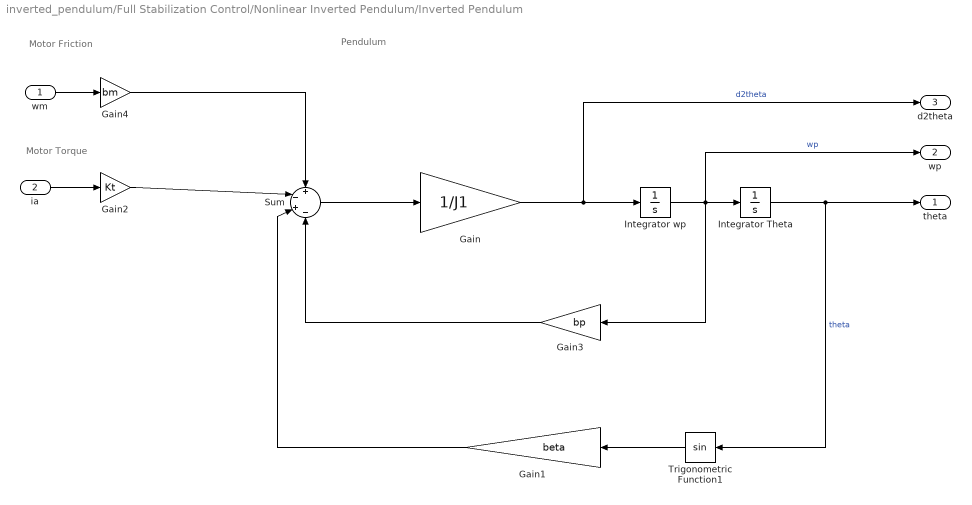
== system inverted_pendulum/Full Stabilization Control/Nonlinear Inverted Pendulum/Inverted Pendulum ==
  note: Pendulum
  note: Motor Friction
  note: Motor Torque
  wm : Inport
  ia : Inport  Port=2
  Gain : Gain  Gain=1/J1
  Gain1 : Gain  Gain=beta
  Gain2 : Gain  Gain=Kt
  Gain3 : Gain  Gain=bp
  Gain4 : Gain  Gain=bm
  Integrator Theta : Integrator  InitialCondition=x0(1)
  Integrator wp : Integrator  InitialCondition=x0(2)
  Sum : Sum  Inputs=+-+-
  Trigonometric Function1 : Trigonometry
  theta : Outport
  wp : Outport  Port=2
  d2theta : Outport  Port=3
  wires:
  Trigonometric Function1/1 -> Gain1/1
  Gain/1 -> d2theta/1, Integrator wp/1  "d2theta"
  Sum/1 -> Gain/1
  Integrator Theta/1 -> Trigonometric Function1/1, theta/1  "theta"
  Integrator wp/1 -> wp/1, Gain3/1, Integrator Theta/1  "wp"
  Gain3/1 -> Sum/4
  Gain1/1 -> Sum/3
  ia/1 -> Gain2/1
  Gain2/1 -> Sum/2
  wm/1 -> Gain4/1
  Gain4/1 -> Sum/1

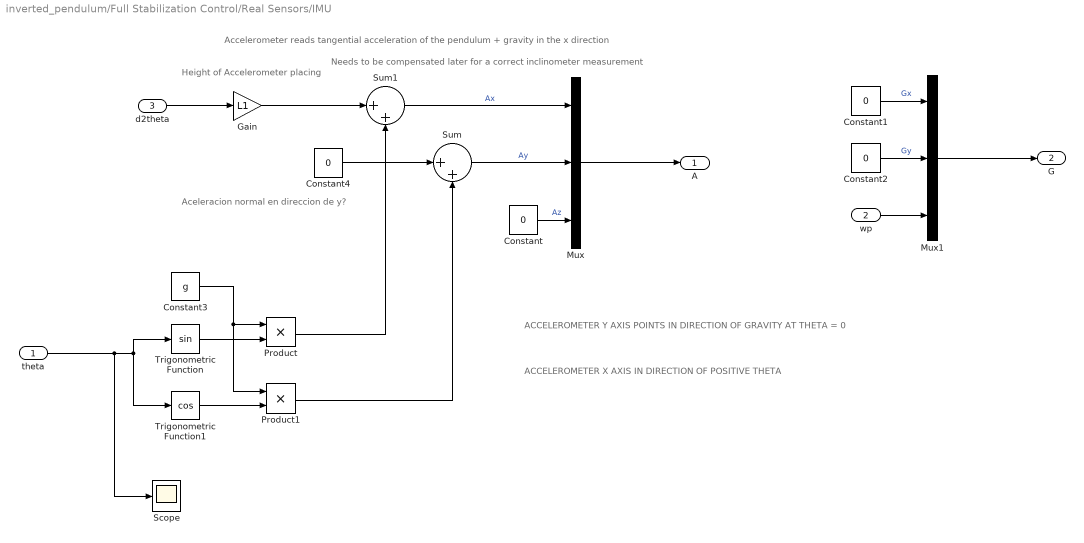
== system inverted_pendulum/Full Stabilization Control/Real Sensors/IMU ==
  note: Aceleracion normal en direccion de y?
  note: Needs to be compensated later for a correct inclinometer measurement
  note: Accelerometer reads tangential acceleration of the pendulum + gravity in the x direction
  note: Height of Accelerometer placing
  note: ACCELEROMETER Y AXIS POINTS IN DIRECTION OF GRAVITY AT THETA = 0
  note: ACCELEROMETER X AXIS IN DIRECTION OF POSITIVE THETA
  theta : Inport
  wp : Inport  Port=2
  d2theta : Inport  Port=3
  Constant{,1..2,4} (4 alike) : Constant  Value=0
  Constant3 : Constant  Value=g
  Gain : Gain  Gain=L1
  Mux : Mux  Inputs=3
  Mux1 : Mux  Inputs=3
  Product : Product
  Product1 : Product
  Scope : Scope
  Sum : Sum  Inputs=|++
  Sum1 : Sum  Inputs=|++
  Trigonometric Function : Trigonometry
  Trigonometric Function1 : Trigonometry  Operator=cos
  A : Outport
  G : Outport  Port=2
  wires:
  Mux/1 -> A/1
  Mux1/1 -> G/1
  Sum/1 -> Mux/2  "Ay"
  Constant/1 -> Mux/3  "Az"
  Sum1/1 -> Mux/1  "Ax"
  Constant2/1 -> Mux1/2  "Gy"
  Constant1/1 -> Mux1/1  "Gx"
  wp/1 -> Mux1/3
  Trigonometric Function/1 -> Product/2
  Trigonometric Function1/1 -> Product1/2
  Constant3/1 -> Product1/1, Product/1
  Product1/1 -> Sum/2
  Product/1 -> Sum1/2
  Constant4/1 -> Sum/1
  theta/1 -> Scope/1, Trigonometric Function1/1, Trigonometric Function/1
  Gain/1 -> Sum1/1
  d2theta/1 -> Gain/1

== system inverted_pendulum/Full Stabilization Control/Real Sensors/Pendulum Encoder ==
  In1 : Inport
  wp : Outport
  wires:
  In1/1 -> wp/1

== system inverted_pendulum/Full Stabilization Control/Real Sensors/Wheel Encoder ==
  In1 : Inport
  wm : Outport
  wires:
  In1/1 -> wm/1

== system inverted_pendulum/Full Swing Up Control/Bang Bang Energy Controller/Energy Calculation ==
  note: Potential Energy
  note: Kinetic Energy
  note: Instant Energy
  note: Energy at the top position
  theta : Inport
  wp : Inport  Port=2
  Constant : Constant
  Constant1 : Constant  Value=wn
  Constant2 : Constant  Value=2
  Divide : Product  Inputs=*/
  Gain : Gain  Gain=1/2
  Square : Math  Operator=square  SaturateOnIntegerOverflow=on
  Sum : Sum  Inputs=|+-
  Sum1 : Sum  Inputs=+++
  Trigonometric Function : Trigonometry  Operator=cos
  Eref-E : Outport
  wires:
  Sum/1 -> Eref-E/1
  Constant2/1 -> Sum/1  "Eref"
  Sum1/1 -> Sum/2  "E"
  Constant/1 -> Sum1/3
  Trigonometric Function/1 -> Sum1/2
  theta/1 -> Trigonometric Function/1  "theta"
  Divide/1 -> Square/1
  wp/1 -> Divide/1  "wp"
  Constant1/1 -> Divide/2  "wn"
  Square/1 -> Gain/1
  Gain/1 -> Sum1/1

== system inverted_pendulum/Full Swing Up Control/Nonlinear Inverted Pendulum/DC Motor + Wheel ==
  note: Wheel
  note: DC Motor
  V : Inport
  Gain : Gain  Gain=1/Jw
  Gain1 : Gain  Gain=bm
  Gain2 : Gain  Gain=Kt
  Gain3 : Gain  Gain=1/La
  Gain4 : Gain  Gain=Ra
  Gain5 : Gain  Gain=Ke
  Integrator ia : Integrator  InitialCondition=x0(4)
  Integrator wm : Integrator  InitialCondition=x0(3)
  Sum : Sum  Inputs=|+-
  Sum1 : Sum  Inputs=|+--
  wm : Outport
  ia : Outport  Port=2
  wires:
  Sum/1 -> Gain/1
  Gain/1 -> Integrator wm/1  "d2phi"
  Integrator wm/1 -> wm/1, Gain1/1, Gain5/1  "wm"
  Gain1/1 -> Sum/2
  Gain2/1 -> Sum/1
  Integrator ia/1 -> ia/1, Gain4/1, Gain2/1  "ia"
  Gain3/1 -> Integrator ia/1  "di/dt"
  Sum1/1 -> Gain3/1
  Gain4/1 -> Sum1/3
  V/1 -> Sum1/1  "V"
  Gain5/1 -> Sum1/2

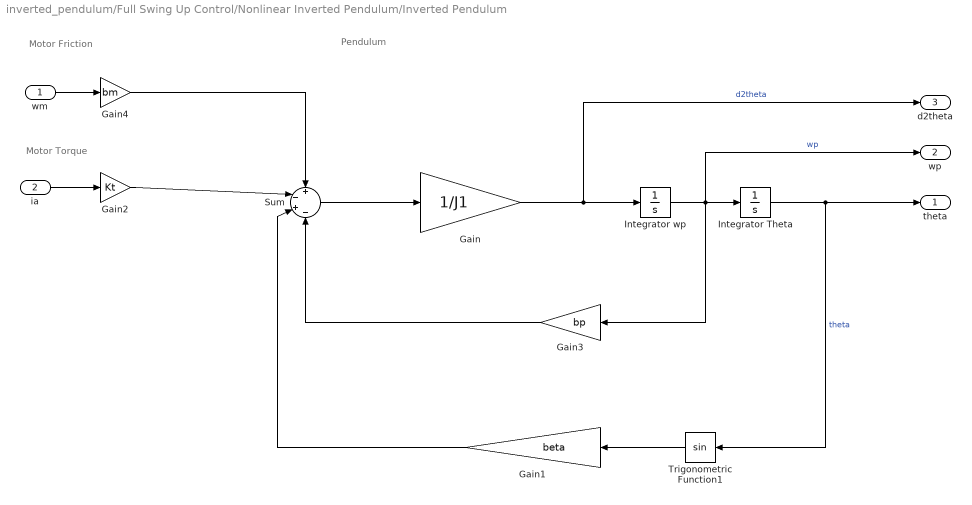
== system inverted_pendulum/Full Swing Up Control/Nonlinear Inverted Pendulum/Inverted Pendulum ==
  note: Pendulum
  note: Motor Friction
  note: Motor Torque
  wm : Inport
  ia : Inport  Port=2
  Gain : Gain  Gain=1/J1
  Gain1 : Gain  Gain=beta
  Gain2 : Gain  Gain=Kt
  Gain3 : Gain  Gain=bp
  Gain4 : Gain  Gain=bm
  Integrator Theta : Integrator  InitialCondition=x0(1)
  Integrator wp : Integrator  InitialCondition=x0(2)
  Sum : Sum  Inputs=+-+-
  Trigonometric Function1 : Trigonometry
  theta : Outport
  wp : Outport  Port=2
  d2theta : Outport  Port=3
  wires:
  Trigonometric Function1/1 -> Gain1/1
  Gain/1 -> d2theta/1, Integrator wp/1  "d2theta"
  Sum/1 -> Gain/1
  Integrator Theta/1 -> Trigonometric Function1/1, theta/1  "theta"
  Integrator wp/1 -> wp/1, Gain3/1, Integrator Theta/1  "wp"
  Gain3/1 -> Sum/4
  Gain1/1 -> Sum/3
  ia/1 -> Gain2/1
  Gain2/1 -> Sum/2
  wm/1 -> Gain4/1
  Gain4/1 -> Sum/1

== system inverted_pendulum/Stabilization Control Full Ideal Sensors/Nonlinear Inverted Pendulum/DC Motor + Wheel ==
  note: Wheel
  note: DC Motor
  V : Inport
  Gain : Gain  Gain=1/Jw
  Gain1 : Gain  Gain=bm
  Gain2 : Gain  Gain=Kt
  Gain3 : Gain  Gain=1/La
  Gain4 : Gain  Gain=Ra
  Gain5 : Gain  Gain=Ke
  Integrator ia : Integrator  InitialCondition=x0(4)
  Integrator wm : Integrator  InitialCondition=x0(3)
  Sum : Sum  Inputs=|+-
  Sum1 : Sum  Inputs=|+--
  wm : Outport
  ia : Outport  Port=2
  wires:
  Sum/1 -> Gain/1
  Gain/1 -> Integrator wm/1  "d2phi"
  Integrator wm/1 -> wm/1, Gain1/1, Gain5/1  "wm"
  Gain1/1 -> Sum/2
  Gain2/1 -> Sum/1
  Integrator ia/1 -> ia/1, Gain4/1, Gain2/1  "ia"
  Gain3/1 -> Integrator ia/1  "di/dt"
  Sum1/1 -> Gain3/1
  Gain4/1 -> Sum1/3
  V/1 -> Sum1/1  "V"
  Gain5/1 -> Sum1/2

== system inverted_pendulum/Stabilization Control Full Ideal Sensors/Nonlinear Inverted Pendulum/Inverted Pendulum ==
  note: Pendulum
  note: Motor Friction
  note: Motor Torque
  wm : Inport
  ia : Inport  Port=2
  Gain : Gain  Gain=1/J1
  Gain1 : Gain  Gain=beta
  Gain2 : Gain  Gain=Kt
  Gain3 : Gain  Gain=bp
  Gain4 : Gain  Gain=bm
  Integrator Theta : Integrator  InitialCondition=x0(1)
  Integrator wp : Integrator  InitialCondition=x0(2)
  Sum : Sum  Inputs=+-+-
  Trigonometric Function1 : Trigonometry
  theta : Outport
  wp : Outport  Port=2
  d2theta : Outport  Port=3
  wires:
  Trigonometric Function1/1 -> Gain1/1
  Gain/1 -> d2theta/1, Integrator wp/1  "d2theta"
  Sum/1 -> Gain/1
  Integrator Theta/1 -> Trigonometric Function1/1, theta/1  "theta"
  Integrator wp/1 -> wp/1, Gain3/1, Integrator Theta/1  "wp"
  Gain3/1 -> Sum/4
  Gain1/1 -> Sum/3
  ia/1 -> Gain2/1
  Gain2/1 -> Sum/2
  wm/1 -> Gain4/1
  Gain4/1 -> Sum/1

== system inverted_pendulum/Stabilization Control Ideal Accelerometer /Nonlinear Inverted Pendulum/DC Motor + Wheel ==
  note: Wheel
  note: DC Motor
  V : Inport
  Gain : Gain  Gain=1/Jw
  Gain1 : Gain  Gain=bm
  Gain2 : Gain  Gain=Kt
  Gain3 : Gain  Gain=1/La
  Gain4 : Gain  Gain=Ra
  Gain5 : Gain  Gain=Ke
  Integrator ia : Integrator  InitialCondition=x0(4)
  Integrator wm : Integrator  InitialCondition=x0(3)
  Sum : Sum  Inputs=|+-
  Sum1 : Sum  Inputs=|+--
  wm : Outport
  ia : Outport  Port=2
  wires:
  Sum/1 -> Gain/1
  Gain/1 -> Integrator wm/1  "d2phi"
  Integrator wm/1 -> wm/1, Gain1/1, Gain5/1  "wm"
  Gain1/1 -> Sum/2
  Gain2/1 -> Sum/1
  Integrator ia/1 -> ia/1, Gain4/1, Gain2/1  "ia"
  Gain3/1 -> Integrator ia/1  "di/dt"
  Sum1/1 -> Gain3/1
  Gain4/1 -> Sum1/3
  V/1 -> Sum1/1  "V"
  Gain5/1 -> Sum1/2

== system inverted_pendulum/Stabilization Control Ideal Accelerometer /Nonlinear Inverted Pendulum/Inverted Pendulum ==
  note: Pendulum
  note: Motor Friction
  note: Motor Torque
  wm : Inport
  ia : Inport  Port=2
  Gain : Gain  Gain=1/J1
  Gain1 : Gain  Gain=beta
  Gain2 : Gain  Gain=Kt
  Gain3 : Gain  Gain=bp
  Gain4 : Gain  Gain=bm
  Integrator Theta : Integrator  InitialCondition=x0(1)
  Integrator wp : Integrator  InitialCondition=x0(2)
  Sum : Sum  Inputs=+-+-
  Trigonometric Function1 : Trigonometry
  theta : Outport
  wp : Outport  Port=2
  d2theta : Outport  Port=3
  wires:
  Trigonometric Function1/1 -> Gain1/1
  Gain/1 -> d2theta/1, Integrator wp/1  "d2theta"
  Sum/1 -> Gain/1
  Integrator Theta/1 -> Trigonometric Function1/1, theta/1  "theta"
  Integrator wp/1 -> wp/1, Gain3/1, Integrator Theta/1  "wp"
  Gain3/1 -> Sum/4
  Gain1/1 -> Sum/3
  ia/1 -> Gain2/1
  Gain2/1 -> Sum/2
  wm/1 -> Gain4/1
  Gain4/1 -> Sum/1

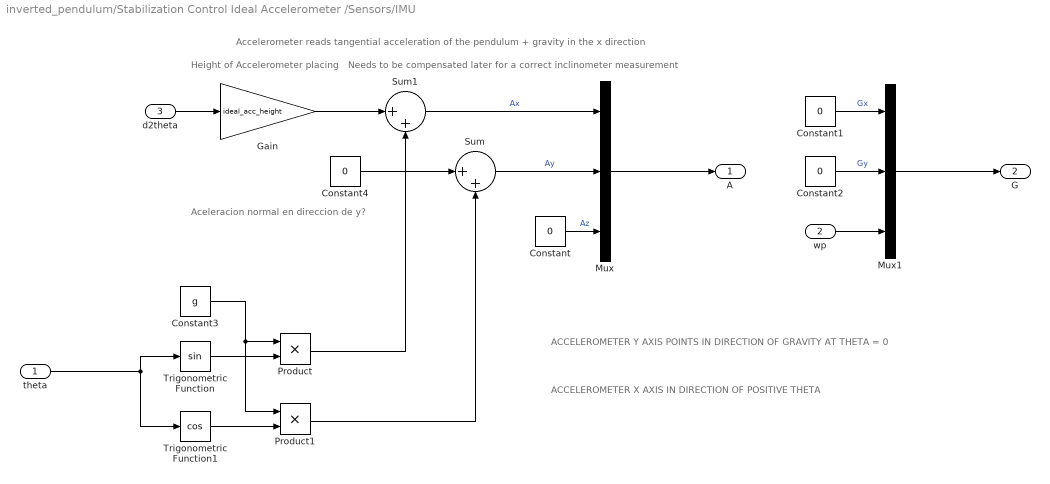
== system inverted_pendulum/Stabilization Control Ideal Accelerometer /Sensors/IMU ==
  note: Aceleracion normal en direccion de y?
  note: Needs to be compensated later for a correct inclinometer measurement
  note: Accelerometer reads tangential acceleration of the pendulum + gravity in the x direction
  note: Height of Accelerometer placing
  note: ACCELEROMETER Y AXIS POINTS IN DIRECTION OF GRAVITY AT THETA = 0
  note: ACCELEROMETER X AXIS IN DIRECTION OF POSITIVE THETA
  theta : Inport
  wp : Inport  Port=2
  d2theta : Inport  Port=3
  Constant{,1..2,4} (4 alike) : Constant  Value=0
  Constant3 : Constant  Value=g
  Gain : Gain  Gain=ideal_acc_height
  Mux : Mux  Inputs=3
  Mux1 : Mux  Inputs=3
  Product : Product
  Product1 : Product
  Sum : Sum  Inputs=|++
  Sum1 : Sum  Inputs=|++
  Trigonometric Function : Trigonometry
  Trigonometric Function1 : Trigonometry  Operator=cos
  A : Outport
  G : Outport  Port=2
  wires:
  Mux/1 -> A/1
  Mux1/1 -> G/1
  Sum/1 -> Mux/2  "Ay"
  Constant/1 -> Mux/3  "Az"
  Sum1/1 -> Mux/1  "Ax"
  Constant2/1 -> Mux1/2  "Gy"
  Constant1/1 -> Mux1/1  "Gx"
  wp/1 -> Mux1/3
  Trigonometric Function/1 -> Product/2
  Trigonometric Function1/1 -> Product1/2
  Constant3/1 -> Product1/1, Product/1
  Product1/1 -> Sum/2
  Product/1 -> Sum1/2
  Constant4/1 -> Sum/1
  theta/1 -> Trigonometric Function1/1, Trigonometric Function/1
  Gain/1 -> Sum1/1
  d2theta/1 -> Gain/1

== system inverted_pendulum/Stabilization Control Real Accelerometer/Nonlinear Inverted Pendulum/DC Motor + Wheel ==
  note: Wheel
  note: DC Motor
  V : Inport
  Gain : Gain  Gain=1/Jw
  Gain1 : Gain  Gain=bm
  Gain2 : Gain  Gain=Kt
  Gain3 : Gain  Gain=1/La
  Gain4 : Gain  Gain=Ra
  Gain5 : Gain  Gain=Ke
  Integrator ia : Integrator  InitialCondition=x0(4)
  Integrator wm : Integrator  InitialCondition=x0(3)
  Sum : Sum  Inputs=|+-
  Sum1 : Sum  Inputs=|+--
  wm : Outport
  ia : Outport  Port=2
  wires:
  Sum/1 -> Gain/1
  Gain/1 -> Integrator wm/1  "d2phi"
  Integrator wm/1 -> wm/1, Gain1/1, Gain5/1  "wm"
  Gain1/1 -> Sum/2
  Gain2/1 -> Sum/1
  Integrator ia/1 -> ia/1, Gain4/1, Gain2/1  "ia"
  Gain3/1 -> Integrator ia/1  "di/dt"
  Sum1/1 -> Gain3/1
  Gain4/1 -> Sum1/3
  V/1 -> Sum1/1  "V"
  Gain5/1 -> Sum1/2

== system inverted_pendulum/Stabilization Control Real Accelerometer/Nonlinear Inverted Pendulum/Inverted Pendulum ==
  note: Pendulum
  note: Motor Friction
  note: Motor Torque
  wm : Inport
  ia : Inport  Port=2
  Gain : Gain  Gain=1/J1
  Gain1 : Gain  Gain=beta
  Gain2 : Gain  Gain=Kt
  Gain3 : Gain  Gain=bp
  Gain4 : Gain  Gain=bm
  Integrator Theta : Integrator  InitialCondition=x0(1)
  Integrator wp : Integrator  InitialCondition=x0(2)
  Sum : Sum  Inputs=+-+-
  Trigonometric Function1 : Trigonometry
  theta : Outport
  wp : Outport  Port=2
  d2theta : Outport  Port=3
  wires:
  Trigonometric Function1/1 -> Gain1/1
  Gain/1 -> d2theta/1, Integrator wp/1  "d2theta"
  Sum/1 -> Gain/1
  Integrator Theta/1 -> Trigonometric Function1/1, theta/1  "theta"
  Integrator wp/1 -> wp/1, Gain3/1, Integrator Theta/1  "wp"
  Gain3/1 -> Sum/4
  Gain1/1 -> Sum/3
  ia/1 -> Gain2/1
  Gain2/1 -> Sum/2
  wm/1 -> Gain4/1
  Gain4/1 -> Sum/1

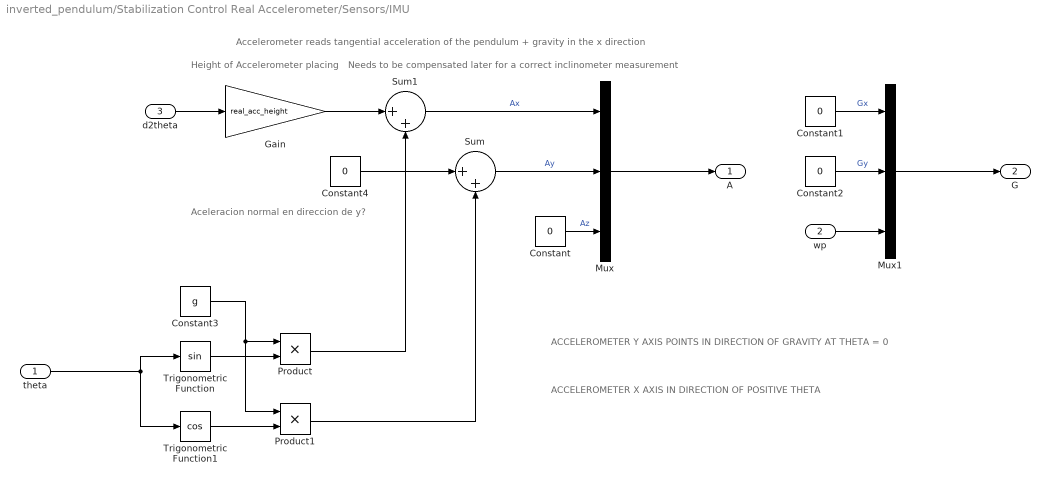
== system inverted_pendulum/Stabilization Control Real Accelerometer/Sensors/IMU ==
  note: Aceleracion normal en direccion de y?
  note: Needs to be compensated later for a correct inclinometer measurement
  note: Accelerometer reads tangential acceleration of the pendulum + gravity in the x direction
  note: Height of Accelerometer placing
  note: ACCELEROMETER Y AXIS POINTS IN DIRECTION OF GRAVITY AT THETA = 0
  note: ACCELEROMETER X AXIS IN DIRECTION OF POSITIVE THETA
  theta : Inport
  wp : Inport  Port=2
  d2theta : Inport  Port=3
  Constant{,1..2,4} (4 alike) : Constant  Value=0
  Constant3 : Constant  Value=g
  Gain : Gain  Gain=real_acc_height
  Mux : Mux  Inputs=3
  Mux1 : Mux  Inputs=3
  Product : Product
  Product1 : Product
  Sum : Sum  Inputs=|++
  Sum1 : Sum  Inputs=|++
  Trigonometric Function : Trigonometry
  Trigonometric Function1 : Trigonometry  Operator=cos
  A : Outport
  G : Outport  Port=2
  wires:
  Mux/1 -> A/1
  Mux1/1 -> G/1
  Sum/1 -> Mux/2  "Ay"
  Constant/1 -> Mux/3  "Az"
  Sum1/1 -> Mux/1  "Ax"
  Constant2/1 -> Mux1/2  "Gy"
  Constant1/1 -> Mux1/1  "Gx"
  wp/1 -> Mux1/3
  Trigonometric Function/1 -> Product/2
  Trigonometric Function1/1 -> Product1/2
  Constant3/1 -> Product1/1, Product/1
  Product1/1 -> Sum/2
  Product/1 -> Sum1/2
  Constant4/1 -> Sum/1
  theta/1 -> Trigonometric Function1/1, Trigonometric Function/1
  Gain/1 -> Sum1/1
  d2theta/1 -> Gain/1
